simulink model "pwm_model"  (R2017a)
settings: Solver=FixedStepAuto  StartTime=0.0  StopTime=10.0  FixedStep=1e-6  RelTol=1e-3
values from neighbouring files (symbols this model uses):
  A = [0, 1; -k/m -b/m]    [mass_1_PWM.m]
  alpha = R/(2*L)    [main.m]    (also in mass_1_PWM.m = 0.5)
  C = 1/model_params(3)    [RLC.m]    (also in main.m)
  max_val = 10    [RLC.m]    (also in main.m = 30; mass_1_PWM.m = 1)
  min_val = -5    [RLC.m]    (also in main.m = -30; mass_1_PWM.m = 0)
  T = 1/f    (= 0.005)    [main.m]    (also in mass_1_PWM.m = 0.05)
  x0 = [0; 0]    [RLC.m]    (also in main.m; mass_1_PWM.m)
undefined symbols (not defined in the file or in its folder): B, D
settings Model: Creator=brunolnetto  LastModifiedBy=brunolnetto

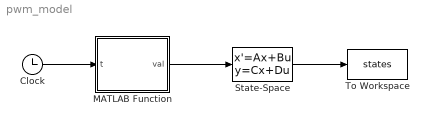
== system pwm_model ==
  Clock : Clock
  MATLAB Function : MATLAB Function  TreatAsAtomicUnit=on
  State-Space : StateSpace  A=A  B=B  C=C  D=D  X0=x0
  To Workspace : ToWorkspace  VariableName=states  SaveFormat=Structure With Time  SampleTime=-1
  wires:
  State-Space/1 -> To Workspace/1
  MATLAB Function/1(val) -> State-Space/1
  Clock/1 -> MATLAB Function/1(t)

== matlab function pwm_model/MATLAB Function ==
  data: t input; val output; max_val parameter; min_val parameter; alpha parameter; T parameter
function val = pwm_signal(t, max_val, min_val, alpha, T)
    persistent t0;
    if(isempty(t0))
        t0 = 0;
    end
    
    if(t == 0)
        t0 = 0;
    end

    if(t - t0 > T)
        t0 = t;
    end

    t_i = t - t0;
    
    if(t_i < alpha*T)
        val = max_val;
    else
        val = min_val;
    end
end
